simulink model "l8Attempt"  (R2016a)
settings: Solver=VariableStepAuto  StartTime=0.0  StopTime=10.0  RelTol=1e-3
settings Model: Creator=Student  LastModifiedBy=Student

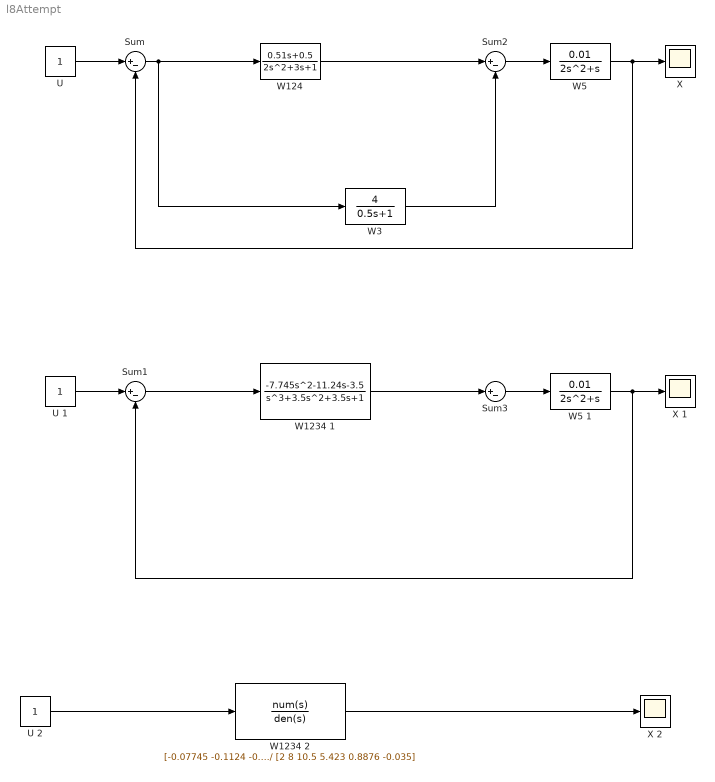
== system l8Attempt ==
  Sum{,1..3} (4 alike) : Sum  Inputs=|+-
  "U " : Constant
  U 1 : Constant
  U 2 : Constant
  W1234 1 : TransferFcn  Numerator=[-7.745 -11.24 -3.5]  Denominator=[1 3.5 3.5 1]
  W1234 2 : TransferFcn  Numerator=[-0.07745 -0.1124 -0.035]  Denominator=[2 8 10.5 5.423 0.8876 -0.035]
  "W124 " : TransferFcn  Numerator=[0.51 0.5]  Denominator=[2 3 1]
  "W3 " : TransferFcn  Numerator=[4]  Denominator=[0.5 1]
  "W5 " : TransferFcn  Numerator=[0.01]  Denominator=[2 1 0]
  W5 1 : TransferFcn  Numerator=[0.01]  Denominator=[2 1 0]
  "X " : Scope
  X 1 : Scope
  X 2 : Scope
  wires:
  "U "/1 -> Sum/1
  Sum/1 -> "W3 "/1, "W124 "/1
  "W124 "/1 -> Sum2/1
  Sum2/1 -> "W5 "/1
  "W5 "/1 -> Sum/2, "X "/1
  "W3 "/1 -> Sum2/2
  U 1/1 -> Sum1/1
  Sum1/1 -> W1234 1/1
  W1234 1/1 -> Sum3/1
  Sum3/1 -> W5 1/1
  W5 1/1 -> Sum1/2, X 1/1
  U 2/1 -> W1234 2/1
  W1234 2/1 -> X 2/1
